simulink model "joint_control_hsiao"  (R2019b)
settings: Solver=ode45  StartTime=0.0  StopTime=t_sim  RelTol=1e-3  EnableMultiTasking=on
values from neighbouring files (symbols this model uses):
  B = 0.0    (= 0)    [or_lab3_params.m]
  d2 = 0.2    [or_lab3_params.m]
  ddtheta_ref = 0    [or_lab3_params.m]
  ddtheta_t = 0    [or_lab3_params.m]
  Delta_Ms = 1    [or_lab3_params.m]
  Delta_theta_1 = pi/4    (= 0.785398163397)    [or_lab3_params.m]
  Delta_theta_2 = pi/4    (= 0.785398163397)    [or_lab3_params.m]
  g = 9.81    [or_lab3_params.m]
  K = 0.5    [or_lab3_params.m]
  m2 = 0.3    [or_lab3_params.m]
  Ms_0 = 0    [or_lab3_params.m]
  mt = 0.3    [or_lab3_params.m]
  R = 0.1    [or_lab3_params.m]
  t_Ms = 1.5    [or_lab3_params.m]
  tau = 1e-4    (= 0.0001)    [or_lab3_params.m]
  theta_ref_0 = 0    [or_lab3_params.m]
  theta_t_1 = 1.0    (= 1)    [or_lab3_params.m]
  theta_t_2 = 2.0    (= 2)    [or_lab3_params.m]
undefined symbols (not defined in the file or in its folder): J, J_n, Kd, Ki, Kp
settings Model: Creator=Damjan  LastModifiedBy=frano
settings DataIOCC: LimitDataPoints=on  SaveFormat=Array  SignalLoggingSaveFormat=ModelDataLogs  ReturnWorkspaceOutputs=off
settings OptimizationCC: ExpressionDepthLimit=2147483647  LifeSpan=inf
settings DebuggingCC: UnderspecifiedInitializationDetection=Classic  MergeDetectMultiDrivingBlocksExec=none  SolverPrmCheckMsg=warning  FcnCallInpInsideContextMsg=warning  StateNameClashWarn=warning  SFUnexpectedBacktrackingDiag=warning  SFNoUnconditionalDefaultTransitionDiag=warning  SFExecutionAtInitializationDiag=none  ArithmeticOperatorsInVariantConditions=warning
settings HardwareCC: ProdBitPerPointer=32  ProdBitPerSizeT=32  ProdBitPerPtrDiffT=32  ProdLargestAtomicFloat=None  ProdIntDivRoundTo=Undefined  ProdEndianess=Unspecified  ProdWordSize=32  ProdHWDeviceType=32-bit Generic
settings ModelReferenceCC: PropagateSignalLabelsOutOfModel=off
settings SFSimCC: SimUseLocalCustomCode=off  CustomCodeUndefinedFunction=UseInterfaceOnly
settings RTWCC: RTWUseLocalCustomCode=off
settings CodeAppCC: StateflowObjectComments=on
settings GRTTargetCC: TargetLangStandard=C89/C90 (ANSI)  GeneratePreprocessorConditionals=Disable all  CombineOutputUpdateFcns=off  GRTInterface=on
settings ConfigComp: CovMetricSettings=dw  CovHtmlReporting=on  CovSaveCumulativeToWorkspaceVar=on  CovSaveSingleToWorkspaceVar=on  CovExternalEMLEnable=off

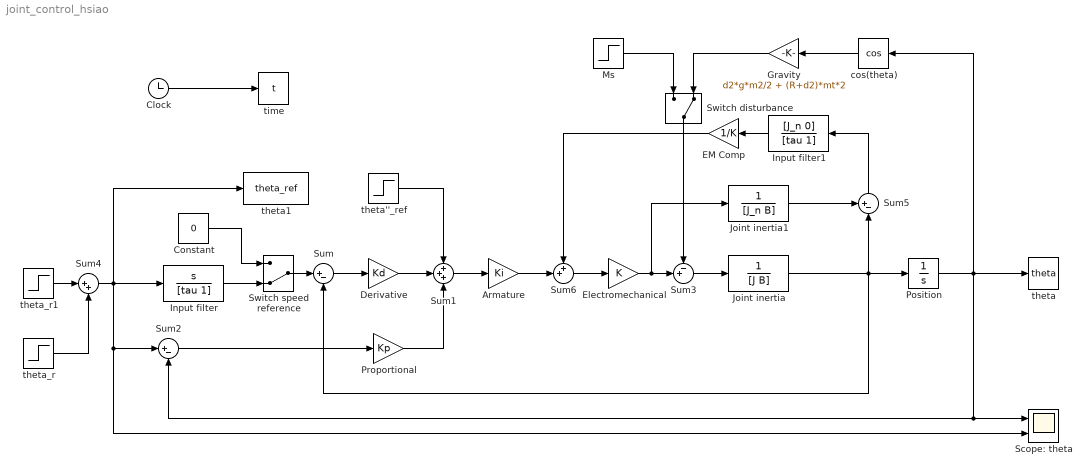
== system joint_control_hsiao ==
  Armature : Gain  Gain=Ki
  Clock : Clock
  Constant : Constant  Value=0
  Derivative : Gain  Gain=Kd
  EM Comp : Gain  Gain=1/K
  Electromechanical : Gain  Gain=K
  Gravity : Gain  Gain=d2*g*m2/2 + (R+d2)*mt*2
  Input filter : TransferFcn  Numerator=[1 0]  Denominator=[tau 1]
  Input filter1 : TransferFcn  Numerator=[J_n 0]  Denominator=[tau 1]
  Joint inertia : TransferFcn  Denominator=[J B]
  Joint inertia1 : TransferFcn  Denominator=[J_n B]
  Ms : Step  Time=t_Ms  Before=Ms_0  After=Ms_0 + Delta_Ms  SampleTime=0
  Position : Integrator
  Proportional : Gain  Gain=Kp
  Scope: theta : Scope  NumInputPorts=2
  Sum : Sum  Inputs=|+-
  Sum1 : Sum  Inputs=+++
  Sum2 : Sum  Inputs=|+-
  Sum3 : Sum  Inputs=-+|
  Sum4 : Sum  Inputs=|++
  Sum5 : Sum  Inputs=+-|
  Sum6 : Sum  Inputs=++|
  Switch disturbance : ManualSwitch  CurrentSetting=0
  Switch speed reference : ManualSwitch  CurrentSetting=0
  cos(theta) : Trigonometry  Operator=cos
  theta : ToWorkspace  VariableName=theta  SampleTime=1/1000
  theta''_ref : Step  Time=ddtheta_t  After=ddtheta_ref  SampleTime=0
  theta1 : ToWorkspace  VariableName=theta_ref  SampleTime=1/1000
  theta_r : Step  Time=theta_t_1  Before=theta_ref_0  After=Delta_theta_1  SampleTime=0
  theta_r1 : Step  Time=theta_t_2  After=Delta_theta_2  SampleTime=0
  time : ToWorkspace  VariableName=t  SampleTime=1/1000
  wires:
  Sum/1 -> Derivative/1
  Sum1/1 -> Armature/1
  Electromechanical/1 -> Joint inertia1/1, Sum3/2
  Position/1 -> cos(theta)/1, theta/1, Sum2/2, Scope: theta/1
  Sum2/1 -> Proportional/1
  Clock/1 -> time/1
  cos(theta)/1 -> Gravity/1
  Ms/1 -> Switch disturbance/1
  Switch disturbance/1 -> Sum3/1
  Gravity/1 -> Switch disturbance/2
  theta_r/1 -> Sum4/2
  theta_r1/1 -> Sum4/1
  Sum4/1 -> theta1/1, Scope: theta/2, Sum2/1, Input filter/1
  Input filter1/1 -> EM Comp/1
  Joint inertia/1 -> Position/1, Sum/2, Sum5/2
  Sum5/1 -> Input filter1/1
  Joint inertia1/1 -> Sum5/1
  Sum3/1 -> Joint inertia/1
  Armature/1 -> Sum6/2
  EM Comp/1 -> Sum6/1
  Sum6/1 -> Electromechanical/1
  Constant/1 -> Switch speed reference/1
  Switch speed reference/1 -> Sum/1
  Input filter/1 -> Switch speed reference/2
  Derivative/1 -> Sum1/2
  Proportional/1 -> Sum1/3
  theta''_ref/1 -> Sum1/1
